simulink model "Preprocessing_Model"  (R2020b)
settings: configuration reference "VLS_Standard_Configuration" (kept outside this file)
libraries: DodecaPreprocessingLib x1
settings Model: DataDictionary=PreprocessingDD.sldd  EnableAccessToBaseWorkspace=off  Creator=sba1  LastModifiedBy=bjothira
settings ConfigSetRef: SourceName=VLS_Standard_Configuration

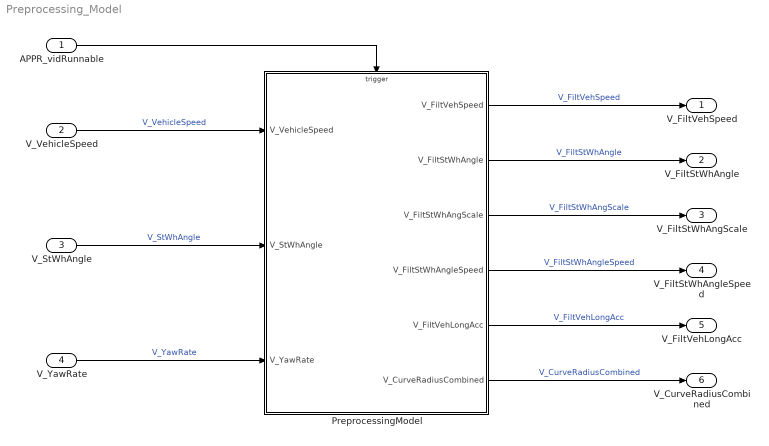
== system Preprocessing_Model ==
  APPR_vidRunnable : Inport  OutputFunctionCall=on
  V_VehicleSpeed : Inport  Port=2
  V_StWhAngle : Inport  Port=3
  V_YawRate : Inport  Port=4
  PreprocessingModel : Subsystem  TreatAsAtomicUnit=on
  V_FiltVehSpeed : Outport  VectorParamsAs1DForOutWhenUnconnected=off
  V_FiltStWhAngle : Outport  Port=2  VectorParamsAs1DForOutWhenUnconnected=off
  V_FiltStWhAngScale : Outport  Port=3  VectorParamsAs1DForOutWhenUnconnected=off
  V_FiltStWhAngleSpeed : Outport  Port=4  VectorParamsAs1DForOutWhenUnconnected=off
  V_FiltVehLongAcc : Outport  Port=5  VectorParamsAs1DForOutWhenUnconnected=off
  V_CurveRadiusCombined : Outport  Port=6  VectorParamsAs1DForOutWhenUnconnected=off
  wires:
  V_YawRate/1 -> PreprocessingModel/3(V_YawRate)  "V_YawRate"
  V_StWhAngle/1 -> PreprocessingModel/2(V_StWhAngle)  "V_StWhAngle"
  V_VehicleSpeed/1 -> PreprocessingModel/1(V_VehicleSpeed)  "V_VehicleSpeed"
  APPR_vidRunnable/1 -> PreprocessingModel/Trigger
  PreprocessingModel/1(V_FiltVehSpeed) -> V_FiltVehSpeed/1  "V_FiltVehSpeed"
  PreprocessingModel/2(V_FiltStWhAngle) -> V_FiltStWhAngle/1  "V_FiltStWhAngle"
  PreprocessingModel/3(V_FiltStWhAngScale) -> V_FiltStWhAngScale/1  "V_FiltStWhAngScale"
  PreprocessingModel/4(V_FiltStWhAngleSpeed) -> V_FiltStWhAngleSpeed/1  "V_FiltStWhAngleSpeed"
  PreprocessingModel/5(V_FiltVehLongAcc) -> V_FiltVehLongAcc/1  "V_FiltVehLongAcc"
  PreprocessingModel/6(V_CurveRadiusCombined) -> V_CurveRadiusCombined/1  "V_CurveRadiusCombined"

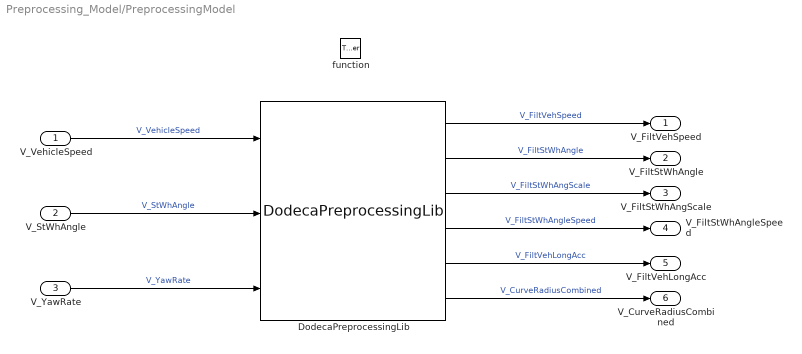
== system Preprocessing_Model/PreprocessingModel ==
  V_VehicleSpeed : Inport
  V_StWhAngle : Inport  Port=2
  V_YawRate : Inport  Port=3
  function : TriggerPort  TriggerType=function-call  VariantControl=Variant
  DodecaPreprocessingLib : DodecaPreprocessingLib/DodecaPreprocessingLib  SystemSampleTime=-1  VariantActivationTime=update diagram  Latency=0  AutoFrameSizeCalculation=off
  V_FiltVehSpeed : Outport  VectorParamsAs1DForOutWhenUnconnected=off
  V_FiltStWhAngle : Outport  Port=2  VectorParamsAs1DForOutWhenUnconnected=off
  V_FiltStWhAngScale : Outport  Port=3  VectorParamsAs1DForOutWhenUnconnected=off
  V_FiltStWhAngleSpeed : Outport  Port=4  VectorParamsAs1DForOutWhenUnconnected=off
  V_FiltVehLongAcc : Outport  Port=5  VectorParamsAs1DForOutWhenUnconnected=off
  V_CurveRadiusCombined : Outport  Port=6  VectorParamsAs1DForOutWhenUnconnected=off
  wires:
  DodecaPreprocessingLib/1 -> V_FiltVehSpeed/1  "V_FiltVehSpeed"
  DodecaPreprocessingLib/2 -> V_FiltStWhAngle/1  "V_FiltStWhAngle"
  DodecaPreprocessingLib/3 -> V_FiltStWhAngScale/1  "V_FiltStWhAngScale"
  DodecaPreprocessingLib/4 -> V_FiltStWhAngleSpeed/1  "V_FiltStWhAngleSpeed"
  DodecaPreprocessingLib/5 -> V_FiltVehLongAcc/1  "V_FiltVehLongAcc"
  DodecaPreprocessingLib/6 -> V_CurveRadiusCombined/1  "V_CurveRadiusCombined"
  V_VehicleSpeed/1 -> DodecaPreprocessingLib/1  "V_VehicleSpeed"
  V_StWhAngle/1 -> DodecaPreprocessingLib/2  "V_StWhAngle"
  V_YawRate/1 -> DodecaPreprocessingLib/3  "V_YawRate"
